simulink model "Ardupilot_PID_3"  (R2022a)
settings: Solver=VariableStepAuto  StartTime=0.0  StopTime=10.0  RelTol=1e-3
libraries: slpidlib x6, simulink x1
settings Model: Creator=rodri  LastModifiedBy=rodri

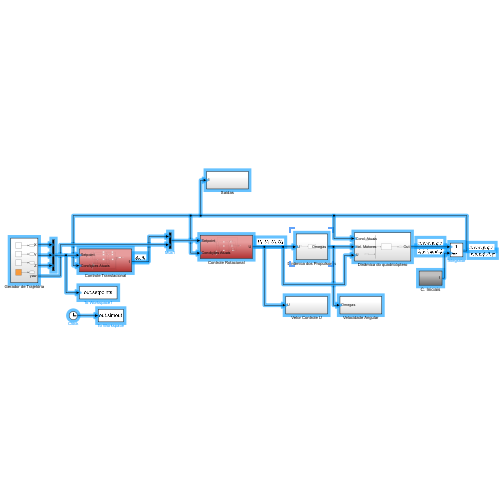
[thumbnail: Simulink's stored preview of the top-level diagram]
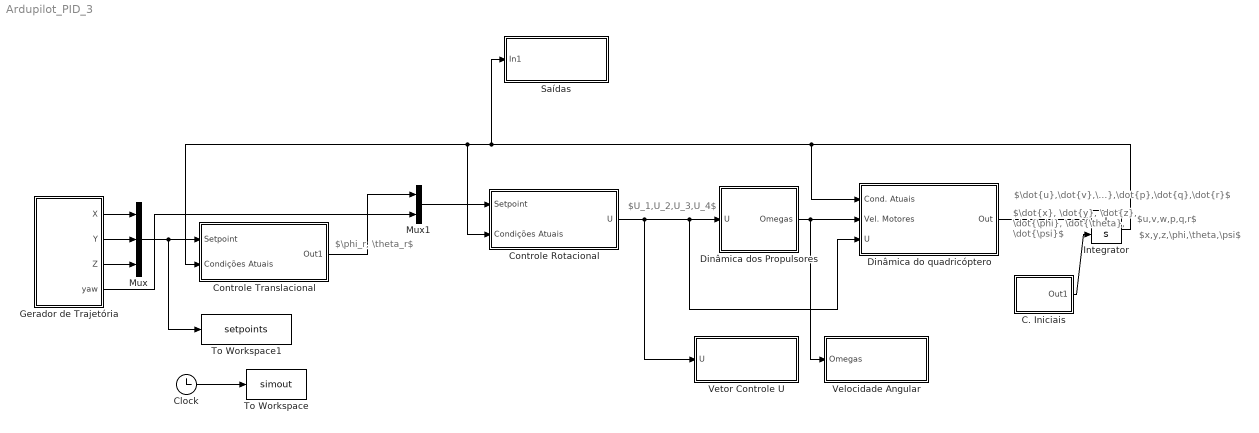
== system Ardupilot_PID_3 ==
  note: $u,v,w,p,q,r$
  note: $\phi_r, \theta_r$
  note: $\dot{u},\dot{v},\dot{w},\dot{p},\dot{q},\dot{r}$
  note: $x,y,z,\phi,\theta,\psi$
  note: $\dot{x}, \dot{y}, \dot{z}, \dot{\phi}, \dot{\theta}, \dot{\psi}$
  note: $U_1,U_2,U_3,U_4$
  C. Iniciais : Subsystem
  Clock : Clock
  Controle Rotacional : Subsystem
  Controle Translacional : Subsystem
  Dinâmica do quadricóptero : Subsystem
  Dinâmica dos Propulsores : Subsystem
  Gerador de Trajetória : Subsystem
  Integrator : Integrator  InitialConditionSource=external
  Mux : Mux  Inputs=3
  Mux1 : Mux  Inputs=2
  Saídas : Subsystem
  To Workspace : ToWorkspace  VariableName=simout  SaveFormat=Structure  SampleTime=-1
  To Workspace1 : ToWorkspace  VariableName=setpoints  SaveFormat=Timeseries  SampleTime=-1
  Velocidade Angular : Subsystem
  Vetor Controle U : Subsystem
  wires:
  Gerador de Trajetória/3(Z) -> Mux/3
  Controle Translacional/1(Out1) -> Mux1/1
  Dinâmica dos Propulsores/1(Omegas) -> Velocidade Angular/1(Omegas), Dinâmica do quadricóptero/2(Vel. Motores)
  Integrator/1 -> Dinâmica do quadricóptero/1(Cond. Atuais), Controle Translacional/2(Condições Atuais), Controle Rotacional/2(Condições Atuais), Saídas/1(In1)
  Gerador de Trajetória/2(Y) -> Mux/2
  C. Iniciais/1(Out1) -> Integrator/2
  Mux1/1 -> Controle Rotacional/1(Setpoint)
  Gerador de Trajetória/1(X) -> Mux/1
  Controle Rotacional/1(U) -> Dinâmica do quadricóptero/3(U), Dinâmica dos Propulsores/1(U), Vetor Controle U/1(U)
  Gerador de Trajetória/4(yaw) -> Mux1/2
  Dinâmica do quadricóptero/1(Out) -> Integrator/1
  Mux/1 -> To Workspace1/1, Controle Translacional/1(Setpoint)
  Clock/1 -> To Workspace/1

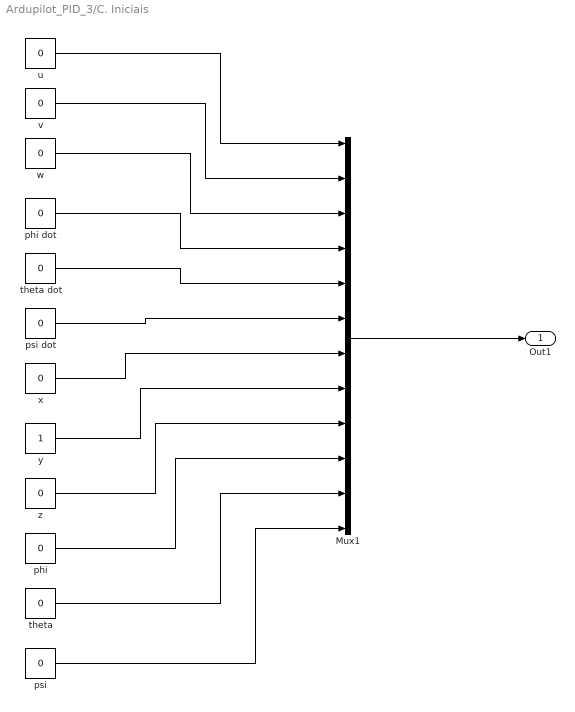
== system Ardupilot_PID_3/C. Iniciais ==
  Mux1 : Mux  Inputs=12
  phi : Constant  Value=0
  phi dot : Constant  Value=0
  psi : Constant  Value=0
  psi dot : Constant  Value=0
  theta : Constant  Value=0
  theta dot : Constant  Value=0
  u : Constant  Value=0
  v : Constant  Value=0
  w : Constant  Value=0
  x : Constant  Value=0
  y : Constant
  z : Constant  Value=0
  Out1 : Outport
  wires:
  u/1 -> Mux1/1
  v/1 -> Mux1/2
  w/1 -> Mux1/3
  phi dot/1 -> Mux1/4
  theta dot/1 -> Mux1/5
  psi dot/1 -> Mux1/6
  x/1 -> Mux1/7
  y/1 -> Mux1/8
  z/1 -> Mux1/9
  phi/1 -> Mux1/10
  theta/1 -> Mux1/11
  psi/1 -> Mux1/12
  Mux1/1 -> Out1/1

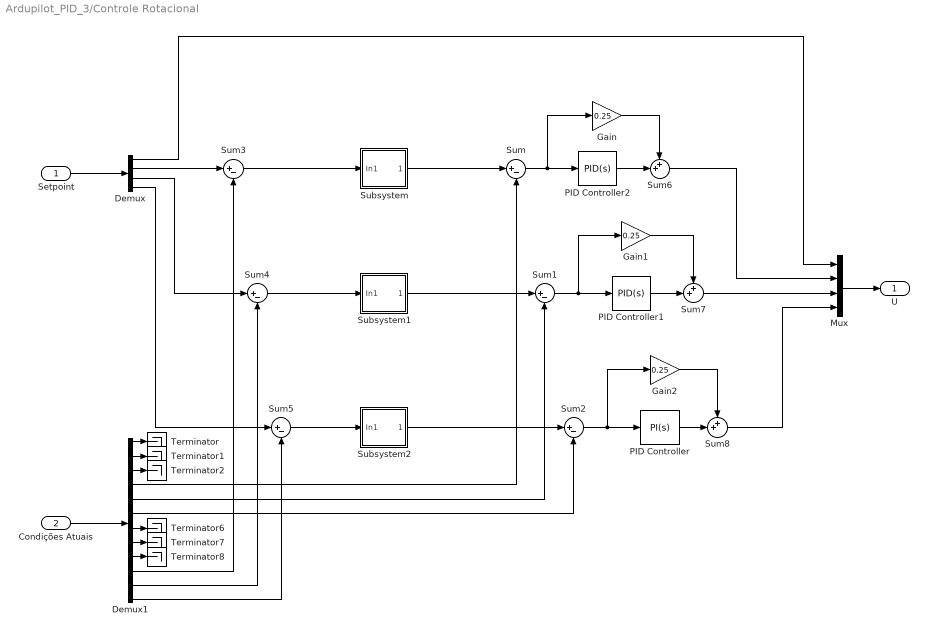
== system Ardupilot_PID_3/Controle Rotacional ==
  Setpoint : Inport
  Condições Atuais : Inport  Port=2
  Demux : Demux
  Demux1 : Demux  Outputs=12
  Gain : Gain  Gain=0.25
  Gain1 : Gain  Gain=0.25
  Gain2 : Gain  Gain=0.25
  Mux : Mux
  PID Controller : slpidlib/PID Controller  Controller=PI  Form=Parallel  TimeDomain=Continuous-time  UseExternalTs=off  SampleTime=-1  IntegratorMethod=Forward Euler  FilterMethod=Forward Euler  ControllerParametersSource=internal  P=0.135  I=0.135  UseKiTs=off  D=-0.00183182159056962  N=2468.24656345106  UseFilter=on  TunerSelectOption=Transfer Function Based (PID Tuner App)  InitialConditionSource=internal  InitialConditionForIntegrator=0  InitialConditionForFilter=0  DifferentiatorICPrevScaledInput=0  ExternalReset=none  TrackingMode=off  Kt=1  LimitOutput=off  SatLimitsSource=internal  UpperSaturationLimit=inf  LowerSaturationLimit=-inf  LinearizeAsGain=on  AntiWindupMode=none  Kb=1  POutMin=[]  POutMax=[]  IOutMin=[]  IOutMax=[]  DOutMin=[]  DOutMax=[]  NOutMin=[]  NOutMax=[]  SumOutMin=[]  SumOutMax=[]  SaturationOutMin=[]  SaturationOutMax=[]  PParamMin=[]  PParamMax=[]  IParamMin=[]  IParamMax=[]  DParamMin=[]  DParamMax=[]  NParamMin=[]  NParamMax=[]  KbParamMin=[]  KbParamMax=[]  KtParamMin=[]  KtParamMax=[]  KbOutMin=[]  KbOutMax=[]  KtOutMin=[]  KtOutMax=[]  IntegratorOutMin=[]  IntegratorOutMax=[]  FilterOutMin=[]  FilterOutMax=[]  SumI1OutMin=[]  SumI1OutMax=[]  SumI2OutMin=[]  SumI2OutMax=[]  SumI3OutMin=[]  SumI3OutMax=[]  SumI4OutMin=[]  SumI4OutMax=[]  SumDOutMin=[]  SumDOutMax=[]  DifferentiatorOutMin=[]  DifferentiatorOutMax=[]  FilterDiffOutCoefMin=[]  FilterDiffOutCoefMax=[]  ReciprocalOutMin=[]  ReciprocalOutMax=[]  SumDenOutMin=[]  SumDenOutMax=[]  SumNumOutMin=[]  SumNumOutMax=[]  DivideOutMin=[]  DivideOutMax=[]  UdiffTsProdOutMin=[]  UdiffTsProdOutMax=[]  NTsProdOutMin=[]  NTsProdOutMax=[]  UintegralTsProdOutMin=[]  UintegralTsProdOutMax=[]  UngainTsProdOutMin=[]  UngainTsProdOutMax=[]  IntegratorContinuousStateAttributes=''  IntegratorStateMustResolveToSignalObject=off  IntegratorRTWStateStorageClass=Auto  FilterContinuousStateAttributes=''  FilterStateMustResolveToSignalObject=off  FilterRTWStateStorageClass=Auto  ParallelPVariant=InternalParameters  IdealPVariant=Disabled  IVariant=InternalParameters  DVariant=Disabled  IntegratorVariant=Continuous  SatVariant=Disabled  AWVariant=Passthrough  PCopyVariant=Disabled  TRVariant=Disabled  FdbkBlocksVariant=Forward  IdealPFdbkVariant=Disabled  SatFdbkVariant=Disabled  DerivativeFilterVariant=Disabled  NVariant=Disabled  NCopyVariant=Disabled_SignalSpec  FilterICVariant=Disabled  IntegratorICVariant=InternalICs  ExternalResetVariant=Disabled  TRSumVariant=Passthrough  SumFdbkVariant=Disabled  SumVariant=Sum_PI  TsampFilterVariant=InternalTs  TsampNgainVariant=Passthrough  TsampIntegralVariant=Passthrough  ExternalSaturationOutDataTypeStr=Inherit: Same as second input  aMode=0
  PID Controller1 : slpidlib/PID Controller  Controller=PID  Form=Parallel  TimeDomain=Continuous-time  UseExternalTs=off  SampleTime=-1  IntegratorMethod=Forward Euler  FilterMethod=Forward Euler  ControllerParametersSource=internal  P=0.135  I=0.135  UseKiTs=off  D=0.0036  N=794.493737497618  UseFilter=on  TunerSelectOption=Transfer Function Based (PID Tuner App)  InitialConditionSource=internal  InitialConditionForIntegrator=0  InitialConditionForFilter=0  DifferentiatorICPrevScaledInput=0  ExternalReset=none  TrackingMode=off  Kt=1  LimitOutput=off  SatLimitsSource=internal  UpperSaturationLimit=inf  LowerSaturationLimit=-inf  LinearizeAsGain=on  AntiWindupMode=none  Kb=1  POutMin=[]  POutMax=[]  IOutMin=[]  IOutMax=[]  DOutMin=[]  DOutMax=[]  NOutMin=[]  NOutMax=[]  SumOutMin=[]  SumOutMax=[]  SaturationOutMin=[]  SaturationOutMax=[]  PParamMin=[]  PParamMax=[]  IParamMin=[]  IParamMax=[]  DParamMin=[]  DParamMax=[]  NParamMin=[]  NParamMax=[]  KbParamMin=[]  KbParamMax=[]  KtParamMin=[]  KtParamMax=[]  KbOutMin=[]  KbOutMax=[]  KtOutMin=[]  KtOutMax=[]  IntegratorOutMin=[]  IntegratorOutMax=[]  FilterOutMin=[]  FilterOutMax=[]  SumI1OutMin=[]  SumI1OutMax=[]  SumI2OutMin=[]  SumI2OutMax=[]  SumI3OutMin=[]  SumI3OutMax=[]  SumI4OutMin=[]  SumI4OutMax=[]  SumDOutMin=[]  SumDOutMax=[]  DifferentiatorOutMin=[]  DifferentiatorOutMax=[]  FilterDiffOutCoefMin=[]  FilterDiffOutCoefMax=[]  ReciprocalOutMin=[]  ReciprocalOutMax=[]  SumDenOutMin=[]  SumDenOutMax=[]  SumNumOutMin=[]  SumNumOutMax=[]  DivideOutMin=[]  DivideOutMax=[]  UdiffTsProdOutMin=[]  UdiffTsProdOutMax=[]  NTsProdOutMin=[]  NTsProdOutMax=[]  UintegralTsProdOutMin=[]  UintegralTsProdOutMax=[]  UngainTsProdOutMin=[]  UngainTsProdOutMax=[]  IntegratorContinuousStateAttributes=''  IntegratorStateMustResolveToSignalObject=off  IntegratorRTWStateStorageClass=Auto  FilterContinuousStateAttributes=''  FilterStateMustResolveToSignalObject=off  FilterRTWStateStorageClass=Auto  ParallelPVariant=InternalParameters  IdealPVariant=Disabled  IVariant=InternalParameters  DVariant=InternalParameters  IntegratorVariant=Continuous  SatVariant=Disabled  AWVariant=Passthrough  PCopyVariant=Disabled  TRVariant=Disabled  FdbkBlocksVariant=Forward  IdealPFdbkVariant=Disabled  SatFdbkVariant=Disabled  DerivativeFilterVariant=ContFilter  NVariant=InternalParameters  NCopyVariant=Disabled  FilterICVariant=InternalICsFilter  IntegratorICVariant=InternalICs  ExternalResetVariant=Disabled  TRSumVariant=Passthrough  SumFdbkVariant=Disabled  SumVariant=Sum_PID  TsampFilterVariant=InternalTs  TsampNgainVariant=Passthrough  TsampIntegralVariant=Passthrough  ExternalSaturationOutDataTypeStr=Inherit: Same as second input  aMode=0
  PID Controller2 : slpidlib/PID Controller  Controller=PID  Form=Parallel  TimeDomain=Continuous-time  UseExternalTs=off  SampleTime=-1  IntegratorMethod=Forward Euler  FilterMethod=Forward Euler  ControllerParametersSource=internal  P=0.135  I=0.135  UseKiTs=off  D=0.0036  N=592.325757045519  UseFilter=on  TunerSelectOption=Transfer Function Based (PID Tuner App)  InitialConditionSource=internal  InitialConditionForIntegrator=0  InitialConditionForFilter=0  DifferentiatorICPrevScaledInput=0  ExternalReset=none  TrackingMode=off  Kt=1  LimitOutput=off  SatLimitsSource=internal  UpperSaturationLimit=inf  LowerSaturationLimit=-inf  LinearizeAsGain=on  AntiWindupMode=none  Kb=1  POutMin=[]  POutMax=[]  IOutMin=[]  IOutMax=[]  DOutMin=[]  DOutMax=[]  NOutMin=[]  NOutMax=[]  SumOutMin=[]  SumOutMax=[]  SaturationOutMin=[]  SaturationOutMax=[]  PParamMin=[]  PParamMax=[]  IParamMin=[]  IParamMax=[]  DParamMin=[]  DParamMax=[]  NParamMin=[]  NParamMax=[]  KbParamMin=[]  KbParamMax=[]  KtParamMin=[]  KtParamMax=[]  KbOutMin=[]  KbOutMax=[]  KtOutMin=[]  KtOutMax=[]  IntegratorOutMin=[]  IntegratorOutMax=[]  FilterOutMin=[]  FilterOutMax=[]  SumI1OutMin=[]  SumI1OutMax=[]  SumI2OutMin=[]  SumI2OutMax=[]  SumI3OutMin=[]  SumI3OutMax=[]  SumI4OutMin=[]  SumI4OutMax=[]  SumDOutMin=[]  SumDOutMax=[]  DifferentiatorOutMin=[]  DifferentiatorOutMax=[]  FilterDiffOutCoefMin=[]  FilterDiffOutCoefMax=[]  ReciprocalOutMin=[]  ReciprocalOutMax=[]  SumDenOutMin=[]  SumDenOutMax=[]  SumNumOutMin=[]  SumNumOutMax=[]  DivideOutMin=[]  DivideOutMax=[]  UdiffTsProdOutMin=[]  UdiffTsProdOutMax=[]  NTsProdOutMin=[]  NTsProdOutMax=[]  UintegralTsProdOutMin=[]  UintegralTsProdOutMax=[]  UngainTsProdOutMin=[]  UngainTsProdOutMax=[]  IntegratorContinuousStateAttributes=''  IntegratorStateMustResolveToSignalObject=off  IntegratorRTWStateStorageClass=Auto  FilterContinuousStateAttributes=''  FilterStateMustResolveToSignalObject=off  FilterRTWStateStorageClass=Auto  ParallelPVariant=InternalParameters  IdealPVariant=Disabled  IVariant=InternalParameters  DVariant=InternalParameters  IntegratorVariant=Continuous  SatVariant=Disabled  AWVariant=Passthrough  PCopyVariant=Disabled  TRVariant=Disabled  FdbkBlocksVariant=Forward  IdealPFdbkVariant=Disabled  SatFdbkVariant=Disabled  DerivativeFilterVariant=ContFilter  NVariant=InternalParameters  NCopyVariant=Disabled  FilterICVariant=InternalICsFilter  IntegratorICVariant=InternalICs  ExternalResetVariant=Disabled  TRSumVariant=Passthrough  SumFdbkVariant=Disabled  SumVariant=Sum_PID  TsampFilterVariant=InternalTs  TsampNgainVariant=Passthrough  TsampIntegralVariant=Passthrough  ExternalSaturationOutDataTypeStr=Inherit: Same as second input  aMode=0
  Subsystem : Subsystem
      mask Display: image('C:\Users\rodri\OneDrive\Imagens\Captura de tela 2025-05-23 002649.PNG'); % Use "Edit Image" on toolstrip to change.
  Subsystem1 : Subsystem
      mask Display: image('C:\Users\rodri\OneDrive\Imagens\Captura de tela 2025-05-23 002649.PNG'); % Use "Edit Image" on toolstrip to change.
  Subsystem2 : Subsystem
      mask Display: image('C:\Users\rodri\OneDrive\Imagens\Captura de tela 2025-05-23 002649.PNG'); % Use "Edit Image" on toolstrip to change.
  Sum{,1..5} (6 alike) : Sum  Inputs=|+-
  Sum6 : Sum  Inputs=++|
  Sum7 : Sum  Inputs=++|
  Sum8 : Sum  Inputs=++|
  Terminator{,1..2,6..8} (6 alike) : Terminator
  U : Outport
  wires:
  Condições Atuais/1 -> Demux1/1
  Demux1/10 -> Sum3/2
  Demux1/12 -> Sum5/2
  Demux1/11 -> Sum4/2
  Mux/1 -> U/1
  Setpoint/1 -> Demux/1
  Demux1/1 -> Terminator/1
  Demux1/2 -> Terminator1/1
  Demux1/3 -> Terminator2/1
  Demux1/4 -> Sum/2
  Demux1/5 -> Sum1/2
  Demux1/6 -> Sum2/2
  Demux1/7 -> Terminator6/1
  Demux1/8 -> Terminator7/1
  Demux1/9 -> Terminator8/1
  Demux/1 -> Mux/1
  Sum/1 -> Gain/1, PID Controller2/1
  Sum1/1 -> Gain1/1, PID Controller1/1
  Sum2/1 -> Gain2/1, PID Controller/1
  Sum5/1 -> Subsystem2/1(In1)
  Sum3/1 -> Subsystem/1(In1)
  Sum4/1 -> Subsystem1/1(In1)
  Demux/2 -> Sum3/1
  Demux/3 -> Sum4/1
  Demux/4 -> Sum5/1
  Subsystem/1(Out1) -> Sum/1
  Subsystem1/1(Out1) -> Sum1/1
  Subsystem2/1(Out1) -> Sum2/1
  PID Controller2/1 -> Sum6/2
  Gain/1 -> Sum6/1
  Sum6/1 -> Mux/2
  Gain1/1 -> Sum7/1
  PID Controller1/1 -> Sum7/2
  Sum7/1 -> Mux/3
  PID Controller/1 -> Sum8/2
  Gain2/1 -> Sum8/1
  Sum8/1 -> Mux/4

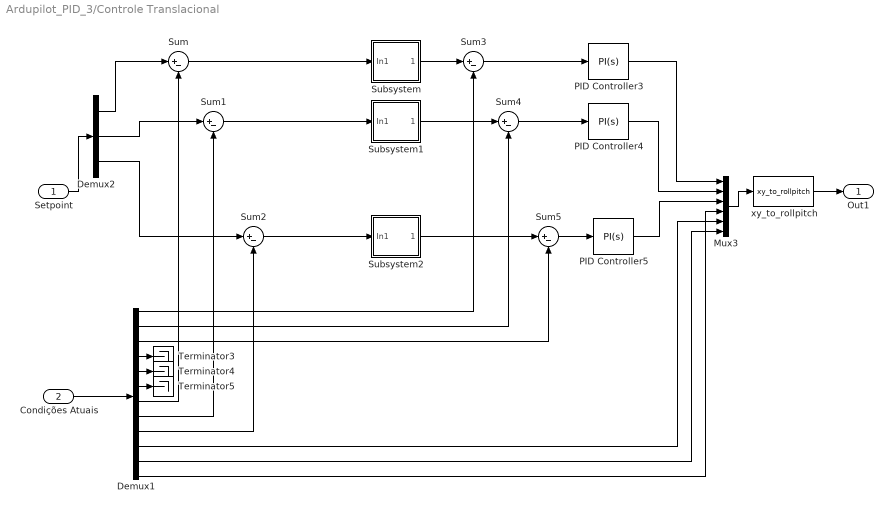
== system Ardupilot_PID_3/Controle Translacional ==
  Setpoint : Inport
  Condições Atuais : Inport  Port=2
  Demux1 : Demux  Outputs=12
  Demux2 : Demux  Outputs=3
  Mux3 : Mux  Inputs=6
  PID Controller3 : slpidlib/PID Controller  Controller=PI  Form=Parallel  TimeDomain=Continuous-time  UseExternalTs=off  SampleTime=-1  IntegratorMethod=Forward Euler  FilterMethod=Forward Euler  ControllerParametersSource=internal  P=1  I=0.5  UseKiTs=off  D=0.5  N=51.8818655440294  UseFilter=on  TunerSelectOption=Transfer Function Based (PID Tuner App)  InitialConditionSource=internal  InitialConditionForIntegrator=0  InitialConditionForFilter=0  DifferentiatorICPrevScaledInput=0  ExternalReset=none  TrackingMode=off  Kt=1  LimitOutput=off  SatLimitsSource=internal  UpperSaturationLimit=inf  LowerSaturationLimit=-inf  LinearizeAsGain=on  AntiWindupMode=none  Kb=1  POutMin=[]  POutMax=[]  IOutMin=[]  IOutMax=[]  DOutMin=[]  DOutMax=[]  NOutMin=[]  NOutMax=[]  SumOutMin=[]  SumOutMax=[]  SaturationOutMin=[]  SaturationOutMax=[]  PParamMin=[]  PParamMax=[]  IParamMin=[]  IParamMax=[]  DParamMin=[]  DParamMax=[]  NParamMin=[]  NParamMax=[]  KbParamMin=[]  KbParamMax=[]  KtParamMin=[]  KtParamMax=[]  KbOutMin=[]  KbOutMax=[]  KtOutMin=[]  KtOutMax=[]  IntegratorOutMin=[]  IntegratorOutMax=[]  FilterOutMin=[]  FilterOutMax=[]  SumI1OutMin=[]  SumI1OutMax=[]  SumI2OutMin=[]  SumI2OutMax=[]  SumI3OutMin=[]  SumI3OutMax=[]  SumI4OutMin=[]  SumI4OutMax=[]  SumDOutMin=[]  SumDOutMax=[]  DifferentiatorOutMin=[]  DifferentiatorOutMax=[]  FilterDiffOutCoefMin=[]  FilterDiffOutCoefMax=[]  ReciprocalOutMin=[]  ReciprocalOutMax=[]  SumDenOutMin=[]  SumDenOutMax=[]  SumNumOutMin=[]  SumNumOutMax=[]  DivideOutMin=[]  DivideOutMax=[]  UdiffTsProdOutMin=[]  UdiffTsProdOutMax=[]  NTsProdOutMin=[]  NTsProdOutMax=[]  UintegralTsProdOutMin=[]  UintegralTsProdOutMax=[]  UngainTsProdOutMin=[]  UngainTsProdOutMax=[]  IntegratorContinuousStateAttributes=''  IntegratorStateMustResolveToSignalObject=off  IntegratorRTWStateStorageClass=Auto  FilterContinuousStateAttributes=''  FilterStateMustResolveToSignalObject=off  FilterRTWStateStorageClass=Auto  ParallelPVariant=InternalParameters  IdealPVariant=Disabled  IVariant=InternalParameters  DVariant=Disabled  IntegratorVariant=Continuous  SatVariant=Disabled  AWVariant=Passthrough  PCopyVariant=Disabled  TRVariant=Disabled  FdbkBlocksVariant=Forward  IdealPFdbkVariant=Disabled  SatFdbkVariant=Disabled  DerivativeFilterVariant=Disabled  NVariant=Disabled  NCopyVariant=Disabled_SignalSpec  FilterICVariant=Disabled  IntegratorICVariant=InternalICs  ExternalResetVariant=Disabled  TRSumVariant=Passthrough  SumFdbkVariant=Disabled  SumVariant=Sum_PI  TsampFilterVariant=InternalTs  TsampNgainVariant=Passthrough  TsampIntegralVariant=Passthrough  ExternalSaturationOutDataTypeStr=Inherit: Same as second input  aMode=0
  PID Controller4 : slpidlib/PID Controller  Controller=PI  Form=Parallel  TimeDomain=Continuous-time  UseExternalTs=off  SampleTime=-1  IntegratorMethod=Forward Euler  FilterMethod=Forward Euler  ControllerParametersSource=internal  P=1  I=0.5  UseKiTs=off  D=1.34953057380817  N=75.9442691323849  UseFilter=on  TunerSelectOption=Transfer Function Based (PID Tuner App)  InitialConditionSource=internal  InitialConditionForIntegrator=0  InitialConditionForFilter=0  DifferentiatorICPrevScaledInput=0  ExternalReset=none  TrackingMode=off  Kt=1  LimitOutput=off  SatLimitsSource=internal  UpperSaturationLimit=inf  LowerSaturationLimit=-inf  LinearizeAsGain=on  AntiWindupMode=none  Kb=1  POutMin=[]  POutMax=[]  IOutMin=[]  IOutMax=[]  DOutMin=[]  DOutMax=[]  NOutMin=[]  NOutMax=[]  SumOutMin=[]  SumOutMax=[]  SaturationOutMin=[]  SaturationOutMax=[]  PParamMin=[]  PParamMax=[]  IParamMin=[]  IParamMax=[]  DParamMin=[]  DParamMax=[]  NParamMin=[]  NParamMax=[]  KbParamMin=[]  KbParamMax=[]  KtParamMin=[]  KtParamMax=[]  KbOutMin=[]  KbOutMax=[]  KtOutMin=[]  KtOutMax=[]  IntegratorOutMin=[]  IntegratorOutMax=[]  FilterOutMin=[]  FilterOutMax=[]  SumI1OutMin=[]  SumI1OutMax=[]  SumI2OutMin=[]  SumI2OutMax=[]  SumI3OutMin=[]  SumI3OutMax=[]  SumI4OutMin=[]  SumI4OutMax=[]  SumDOutMin=[]  SumDOutMax=[]  DifferentiatorOutMin=[]  DifferentiatorOutMax=[]  FilterDiffOutCoefMin=[]  FilterDiffOutCoefMax=[]  ReciprocalOutMin=[]  ReciprocalOutMax=[]  SumDenOutMin=[]  SumDenOutMax=[]  SumNumOutMin=[]  SumNumOutMax=[]  DivideOutMin=[]  DivideOutMax=[]  UdiffTsProdOutMin=[]  UdiffTsProdOutMax=[]  NTsProdOutMin=[]  NTsProdOutMax=[]  UintegralTsProdOutMin=[]  UintegralTsProdOutMax=[]  UngainTsProdOutMin=[]  UngainTsProdOutMax=[]  IntegratorContinuousStateAttributes=''  IntegratorStateMustResolveToSignalObject=off  IntegratorRTWStateStorageClass=Auto  FilterContinuousStateAttributes=''  FilterStateMustResolveToSignalObject=off  FilterRTWStateStorageClass=Auto  ParallelPVariant=InternalParameters  IdealPVariant=Disabled  IVariant=InternalParameters  DVariant=Disabled  IntegratorVariant=Continuous  SatVariant=Disabled  AWVariant=Passthrough  PCopyVariant=Disabled  TRVariant=Disabled  FdbkBlocksVariant=Forward  IdealPFdbkVariant=Disabled  SatFdbkVariant=Disabled  DerivativeFilterVariant=Disabled  NVariant=Disabled  NCopyVariant=Disabled_SignalSpec  FilterICVariant=Disabled  IntegratorICVariant=InternalICs  ExternalResetVariant=Disabled  TRSumVariant=Passthrough  SumFdbkVariant=Disabled  SumVariant=Sum_PI  TsampFilterVariant=InternalTs  TsampNgainVariant=Passthrough  TsampIntegralVariant=Passthrough  ExternalSaturationOutDataTypeStr=Inherit: Same as second input  aMode=0
  PID Controller5 : slpidlib/PID Controller  Controller=PI  Form=Parallel  TimeDomain=Continuous-time  UseExternalTs=off  SampleTime=-1  IntegratorMethod=Forward Euler  FilterMethod=Forward Euler  ControllerParametersSource=internal  P=5  I=2  UseKiTs=off  D=-0.163263956385678  N=128.938404253656  UseFilter=on  TunerSelectOption=Transfer Function Based (PID Tuner App)  InitialConditionSource=internal  InitialConditionForIntegrator=0  InitialConditionForFilter=0  DifferentiatorICPrevScaledInput=0  ExternalReset=none  TrackingMode=off  Kt=1  LimitOutput=off  SatLimitsSource=internal  UpperSaturationLimit=inf  LowerSaturationLimit=-inf  LinearizeAsGain=on  AntiWindupMode=none  Kb=1  POutMin=[]  POutMax=[]  IOutMin=[]  IOutMax=[]  DOutMin=[]  DOutMax=[]  NOutMin=[]  NOutMax=[]  SumOutMin=[]  SumOutMax=[]  SaturationOutMin=[]  SaturationOutMax=[]  PParamMin=[]  PParamMax=[]  IParamMin=[]  IParamMax=[]  DParamMin=[]  DParamMax=[]  NParamMin=[]  NParamMax=[]  KbParamMin=[]  KbParamMax=[]  KtParamMin=[]  KtParamMax=[]  KbOutMin=[]  KbOutMax=[]  KtOutMin=[]  KtOutMax=[]  IntegratorOutMin=[]  IntegratorOutMax=[]  FilterOutMin=[]  FilterOutMax=[]  SumI1OutMin=[]  SumI1OutMax=[]  SumI2OutMin=[]  SumI2OutMax=[]  SumI3OutMin=[]  SumI3OutMax=[]  SumI4OutMin=[]  SumI4OutMax=[]  SumDOutMin=[]  SumDOutMax=[]  DifferentiatorOutMin=[]  DifferentiatorOutMax=[]  FilterDiffOutCoefMin=[]  FilterDiffOutCoefMax=[]  ReciprocalOutMin=[]  ReciprocalOutMax=[]  SumDenOutMin=[]  SumDenOutMax=[]  SumNumOutMin=[]  SumNumOutMax=[]  DivideOutMin=[]  DivideOutMax=[]  UdiffTsProdOutMin=[]  UdiffTsProdOutMax=[]  NTsProdOutMin=[]  NTsProdOutMax=[]  UintegralTsProdOutMin=[]  UintegralTsProdOutMax=[]  UngainTsProdOutMin=[]  UngainTsProdOutMax=[]  IntegratorContinuousStateAttributes=''  IntegratorStateMustResolveToSignalObject=off  IntegratorRTWStateStorageClass=Auto  FilterContinuousStateAttributes=''  FilterStateMustResolveToSignalObject=off  FilterRTWStateStorageClass=Auto  ParallelPVariant=InternalParameters  IdealPVariant=Disabled  IVariant=InternalParameters  DVariant=Disabled  IntegratorVariant=Continuous  SatVariant=Disabled  AWVariant=Passthrough  PCopyVariant=Disabled  TRVariant=Disabled  FdbkBlocksVariant=Forward  IdealPFdbkVariant=Disabled  SatFdbkVariant=Disabled  DerivativeFilterVariant=Disabled  NVariant=Disabled  NCopyVariant=Disabled_SignalSpec  FilterICVariant=Disabled  IntegratorICVariant=InternalICs  ExternalResetVariant=Disabled  TRSumVariant=Passthrough  SumFdbkVariant=Disabled  SumVariant=Sum_PI  TsampFilterVariant=InternalTs  TsampNgainVariant=Passthrough  TsampIntegralVariant=Passthrough  ExternalSaturationOutDataTypeStr=Inherit: Same as second input  aMode=0
  Subsystem : Subsystem
      mask Display: image('C:\Users\rodri\OneDrive\Imagens\Captura de tela 2025-05-23 002649.PNG'); % Use "Edit Image" on toolstrip to change.
  Subsystem1 : Subsystem
      mask Display: image('C:\Users\rodri\OneDrive\Imagens\Captura de tela 2025-05-23 002649.PNG'); % Use "Edit Image" on toolstrip to change.
  Subsystem2 : Subsystem
      mask Display: image('C:\Users\rodri\OneDrive\Imagens\Captura de tela 2025-05-23 002649.PNG'); % Use "Edit Image" on toolstrip to change.
  Sum{,1..5} (6 alike) : Sum  Inputs=|+-
  Terminator3 : Terminator
  Terminator4 : Terminator
  Terminator5 : Terminator
  xy_to_rollpitch : MATLABFcn  MATLABFcn=xy_to_rollpitch  OutputDimensions=3
  Out1 : Outport
  wires:
  Demux1/10 -> Mux3/5
  Mux3/1 -> xy_to_rollpitch/1
  xy_to_rollpitch/1 -> Out1/1
  Demux2/2 -> Sum1/1
  Setpoint/1 -> Demux2/1
  Demux1/11 -> Mux3/6
  Demux1/12 -> Mux3/4
  Demux1/8 -> Sum1/2
  Demux1/1 -> Sum3/2
  Demux1/2 -> Sum4/2
  Demux1/6 -> Terminator5/1
  Demux1/4 -> Terminator3/1
  Condições Atuais/1 -> Demux1/1
  Demux1/5 -> Terminator4/1
  Demux1/3 -> Sum5/2
  Demux1/7 -> Sum/2
  Sum/1 -> Subsystem/1(In1)
  Demux2/1 -> Sum/1
  Sum1/1 -> Subsystem1/1(In1)
  Demux2/3 -> Sum2/1
  Sum2/1 -> Subsystem2/1(In1)
  Demux1/9 -> Sum2/2
  Sum3/1 -> PID Controller3/1
  Sum4/1 -> PID Controller4/1
  Sum5/1 -> PID Controller5/1
  Subsystem/1(Out1) -> Sum3/1
  Subsystem1/1(Out1) -> Sum4/1
  PID Controller3/1 -> Mux3/1
  PID Controller4/1 -> Mux3/2
  PID Controller5/1 -> Mux3/3
  Subsystem2/1(Out1) -> Sum5/1

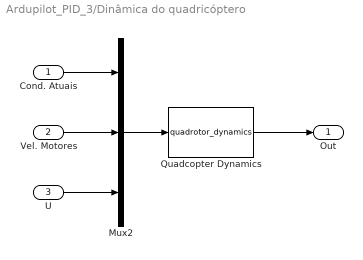
== system Ardupilot_PID_3/Dinâmica do quadricóptero ==
  Cond. Atuais : Inport
  Vel. Motores : Inport  Port=2
  U : Inport  Port=3
  Mux2 : Mux  Inputs=3
  Quadcopter Dynamics : MATLABFcn  MATLABFcn=quadrotor_dynamics  OutputDimensions=12  OutputSignalType=real
  Out : Outport
  wires:
  Mux2/1 -> Quadcopter Dynamics/1
  Cond. Atuais/1 -> Mux2/1
  Vel. Motores/1 -> Mux2/2
  U/1 -> Mux2/3
  Quadcopter Dynamics/1 -> Out/1

== system Ardupilot_PID_3/Dinâmica dos Propulsores ==
  U : Inport
  Rotor Dynamics : MATLABFcn  MATLABFcn=rotor_dynamics  OutputDimensions=4  OutputSignalType=real
  Omegas : Outport
  wires:
  U/1 -> Rotor Dynamics/1
  Rotor Dynamics/1 -> Omegas/1

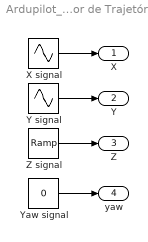
== system Ardupilot_PID_3/Gerador de Trajetória ==
  X signal : Sin  Frequency=2*pi/10  SampleTime=0
  Y signal : Sin  Frequency=2*pi/10  Phase=pi/2  SampleTime=0
  Yaw signal : Constant  Value=0
  Z signal : simulink/Sources/Ramp  slope=0.1  start=0  InitialOutput=0
  X : Outport
  Y : Outport  Port=2
  Z : Outport  Port=3
  yaw : Outport  Port=4
  wires:
  X signal/1 -> X/1
  Y signal/1 -> Y/1
  Z signal/1 -> Z/1
  Yaw signal/1 -> yaw/1

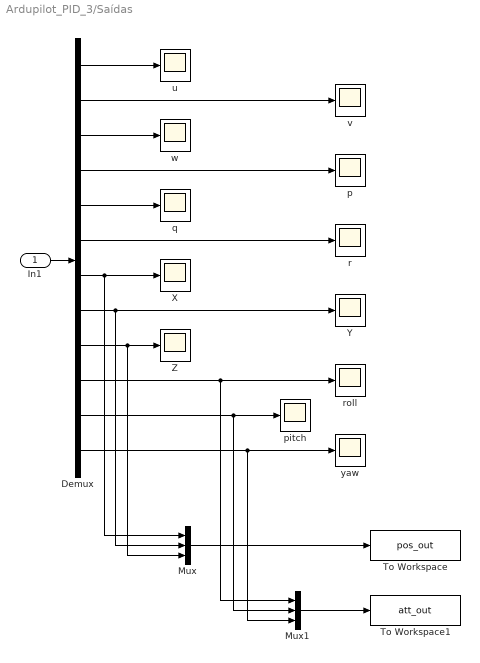
== system Ardupilot_PID_3/Saídas ==
  In1 : Inport
  Demux : Demux  Outputs=12
  Mux : Mux  Inputs=3
  Mux1 : Mux  Inputs=3
  To Workspace : ToWorkspace  VariableName=pos_out  SaveFormat=Timeseries  SampleTime=-1
  To Workspace1 : ToWorkspace  VariableName=att_out  SaveFormat=Timeseries  SampleTime=-1
  X : Scope
  Y : Scope
  Z : Scope
  p : Scope
  pitch : Scope
  q : Scope
  r : Scope
  roll : Scope
  u : Scope
  v : Scope
  w : Scope
  yaw : Scope
  wires:
  In1/1 -> Demux/1
  Demux/1 -> u/1
  Demux/2 -> v/1
  Demux/3 -> w/1
  Demux/4 -> p/1
  Demux/5 -> q/1
  Demux/6 -> r/1
  Demux/7 -> X/1, Mux/1
  Demux/8 -> Mux/2, Y/1
  Demux/10 -> Mux1/1, roll/1
  Demux/11 -> Mux1/2, pitch/1
  Mux/1 -> To Workspace/1
  Mux1/1 -> To Workspace1/1
  Demux/12 -> Mux1/3, yaw/1
  Demux/9 -> Z/1, Mux/3

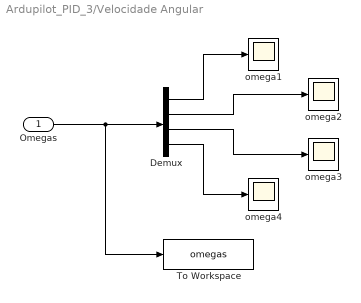
== system Ardupilot_PID_3/Velocidade Angular ==
  Omegas : Inport
  Demux : Demux
  To Workspace : ToWorkspace  VariableName=omegas  SaveFormat=Timeseries  SampleTime=-1
  omega{1..4} (4 alike) : Scope
  wires:
  Demux/4 -> omega4/1
  Demux/3 -> omega3/1
  Demux/2 -> omega2/1
  Demux/1 -> omega1/1
  Omegas/1 -> To Workspace/1, Demux/1

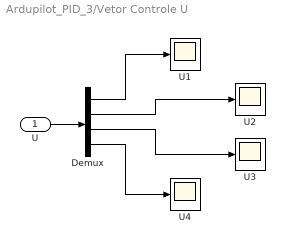
== system Ardupilot_PID_3/Vetor Controle U ==
  U : Inport
  Demux : Demux
  U{1..4} (4 alike) : Scope
  wires:
  U/1 -> Demux/1
  Demux/1 -> U1/1
  Demux/2 -> U2/1
  Demux/3 -> U3/1
  Demux/4 -> U4/1

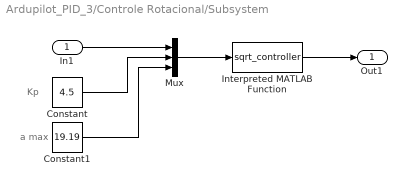
== system Ardupilot_PID_3/Controle Rotacional/Subsystem ==
  note: a max
  note: Kp
  In1 : Inport
  Constant : Constant  Value=4.5
  Constant1 : Constant  Value=19.19
  Interpreted MATLAB Function : MATLABFcn  MATLABFcn=sqrt_controller
  Mux : Mux  Inputs=3
  Out1 : Outport
  wires:
  In1/1 -> Mux/1
  Constant/1 -> Mux/2
  Constant1/1 -> Mux/3
  Mux/1 -> Interpreted MATLAB Function/1
  Interpreted MATLAB Function/1 -> Out1/1

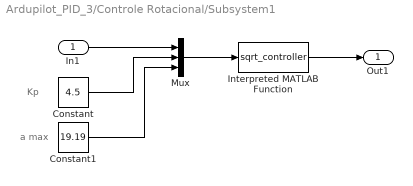
== system Ardupilot_PID_3/Controle Rotacional/Subsystem1 ==
  note: Kp
  note: a max
  In1 : Inport
  Constant : Constant  Value=4.5
  Constant1 : Constant  Value=19.19
  Interpreted MATLAB Function : MATLABFcn  MATLABFcn=sqrt_controller
  Mux : Mux  Inputs=3
  Out1 : Outport
  wires:
  In1/1 -> Mux/1
  Constant/1 -> Mux/2
  Constant1/1 -> Mux/3
  Mux/1 -> Interpreted MATLAB Function/1
  Interpreted MATLAB Function/1 -> Out1/1

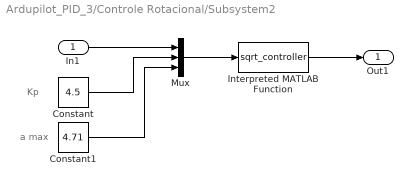
== system Ardupilot_PID_3/Controle Rotacional/Subsystem2 ==
  note: Kp
  note: a max
  In1 : Inport
  Constant : Constant  Value=4.5
  Constant1 : Constant  Value=4.71
  Interpreted MATLAB Function : MATLABFcn  MATLABFcn=sqrt_controller
  Mux : Mux  Inputs=3
  Out1 : Outport
  wires:
  In1/1 -> Mux/1
  Constant/1 -> Mux/2
  Constant1/1 -> Mux/3
  Mux/1 -> Interpreted MATLAB Function/1
  Interpreted MATLAB Function/1 -> Out1/1

== system Ardupilot_PID_3/Controle Translacional/Subsystem ==
  note: Kp
  note: a max
  In1 : Inport
  Constant : Constant
  Constant1 : Constant  Value=5
  Interpreted MATLAB Function : MATLABFcn  MATLABFcn=sqrt_controller
  Mux : Mux  Inputs=3
  Out1 : Outport
  wires:
  In1/1 -> Mux/1
  Constant/1 -> Mux/2
  Constant1/1 -> Mux/3
  Mux/1 -> Interpreted MATLAB Function/1
  Interpreted MATLAB Function/1 -> Out1/1

== system Ardupilot_PID_3/Controle Translacional/Subsystem1 ==
  note: Kp
  note: a max
  In1 : Inport
  Constant : Constant
  Constant1 : Constant  Value=5
  Interpreted MATLAB Function : MATLABFcn  MATLABFcn=sqrt_controller
  Mux : Mux  Inputs=3
  Out1 : Outport
  wires:
  In1/1 -> Mux/1
  Constant/1 -> Mux/2
  Constant1/1 -> Mux/3
  Mux/1 -> Interpreted MATLAB Function/1
  Interpreted MATLAB Function/1 -> Out1/1

== system Ardupilot_PID_3/Controle Translacional/Subsystem2 ==
  note: Kp
  note: a max
  In1 : Inport
  Constant : Constant
  Constant1 : Constant
  Interpreted MATLAB Function : MATLABFcn  MATLABFcn=sqrt_controller
  Mux : Mux  Inputs=3
  Out1 : Outport
  wires:
  In1/1 -> Mux/1
  Constant/1 -> Mux/2
  Constant1/1 -> Mux/3
  Mux/1 -> Interpreted MATLAB Function/1
  Interpreted MATLAB Function/1 -> Out1/1
